simulink library "Px4Library"  (R2015b)
settings: Solver=VariableStepAuto  StartTime=0.0  StopTime=10.0  RelTol=1e-3
undefined symbols (not defined in the file): armed, ctrl_state, INIT_PARAM_VECTOR, mpc_att_sp, mpc_ctrl_state, mpc_manual, mpc_pos_sp_triplet, mpc_vehicle_land_detected, mpc_vehicle_status, v_att_sp, v_control_mode
libraries: simulink x4
(part 7 of 7)

== matlab function Px4Library/attitude_estimator_q/attitude_estimator_q ==
  data: time input; selfVecIn input; selfVecOut output; Q_SAMPLING_PERIOD parameter
function selfVecOut  = qMain( time, selfVecIn, Q_SAMPLING_PERIOD )
%#codegen
	self = DecodeSelf( selfVecIn );
	self = AttitudeEstimatorQ( self, time*1e6 + 149988524 );
	selfVecOut = EncodeSelf( self );
end

function self = DecodeSelf( selfVecIn )
	% Variable assignment
	                           self.acc_comp        = selfVecIn(  1);
	                              self.accel        = zeros( 3, 1);
	                              self.accel( 1, 1) = selfVecIn(  2);
	                              self.accel( 2, 1) = selfVecIn(  3);
	                              self.accel( 3, 1) = selfVecIn(  4);
	    self.airspeed.indicated_airspeed_m_s        = selfVecIn(  5);
	                 self.airspeed.timestamp        = selfVecIn(  6);
	                   self.airspeed.updated        = selfVecIn(  7);
	                      self.airspeed_mode        = selfVecIn(  8);
	self.airspeed_sub.indicated_airspeed_m_s        = selfVecIn(  9);
	             self.airspeed_sub.timestamp        = selfVecIn( 10);
	               self.airspeed_sub.updated        = selfVecIn( 11);
	                  self.att_pub.timestamp        = selfVecIn( 12);
	                  self.att_pub.rollspeed        = selfVecIn( 13);
	                 self.att_pub.pitchspeed        = selfVecIn( 14);
	                   self.att_pub.yawspeed        = selfVecIn( 15);
	                          self.att_pub.q        = zeros( 4, 1);
	                          self.att_pub.q( 1, 1) = selfVecIn( 16);
	                          self.att_pub.q( 2, 1) = selfVecIn( 17);
	                          self.att_pub.q( 3, 1) = selfVecIn( 18);
	                          self.att_pub.q( 4, 1) = selfVecIn( 19);
	                           self.bias_max        = selfVecIn( 20);
	                       self.control_task        = selfVecIn( 21);
	           self.ctrl_state_pub.timestamp        = selfVecIn( 22);
	                   self.ctrl_state_pub.q        = zeros( 4, 1);
	                   self.ctrl_state_pub.q( 1, 1) = selfVecIn( 23);
	                   self.ctrl_state_pub.q( 2, 1) = selfVecIn( 24);
	                   self.ctrl_state_pub.q( 3, 1) = selfVecIn( 25);
	                   self.ctrl_state_pub.q( 4, 1) = selfVecIn( 26);
	               self.ctrl_state_pub.x_acc        = selfVecIn( 27);
	               self.ctrl_state_pub.y_acc        = selfVecIn( 28);
	               self.ctrl_state_pub.z_acc        = selfVecIn( 29);
	           self.ctrl_state_pub.roll_rate        = selfVecIn( 30);
	          self.ctrl_state_pub.pitch_rate        = selfVecIn( 31);
	            self.ctrl_state_pub.yaw_rate        = selfVecIn( 32);
	      self.ctrl_state_pub.roll_rate_bias        = selfVecIn( 33);
	     self.ctrl_state_pub.pitch_rate_bias        = selfVecIn( 34);
	       self.ctrl_state_pub.yaw_rate_bias        = selfVecIn( 35);
	      self.ctrl_state_pub.airspeed_valid        = selfVecIn( 36);
	            self.ctrl_state_pub.airspeed        = selfVecIn( 37);
	                          self.data_good        = selfVecIn( 38);
	                             self.dt_max        = selfVecIn( 39);
	                       self.ext_hdg_good        = selfVecIn( 40);
	                       self.ext_hdg_mode        = selfVecIn( 41);
	             self.global_pos_sub.updated        = selfVecIn( 42);
	                 self.global_pos_sub.eph        = selfVecIn( 43);
	                 self.global_pos_sub.lat        = selfVecIn( 44);
	                 self.global_pos_sub.lon        = selfVecIn( 45);
	           self.global_pos_sub.timestamp        = selfVecIn( 46);
	               self.global_pos_sub.vel_d        = selfVecIn( 47);
	               self.global_pos_sub.vel_e        = selfVecIn( 48);
	               self.global_pos_sub.vel_n        = selfVecIn( 49);
	                       self.gpos.updated        = selfVecIn( 50);
	                           self.gpos.eph        = selfVecIn( 51);
	                           self.gpos.lat        = selfVecIn( 52);
	                           self.gpos.lon        = selfVecIn( 53);
	                     self.gpos.timestamp        = selfVecIn( 54);
	                         self.gpos.vel_d        = selfVecIn( 55);
	                         self.gpos.vel_e        = selfVecIn( 56);
	                         self.gpos.vel_n        = selfVecIn( 57);
	                               self.gyro        = zeros( 3, 1);
	                               self.gyro( 1, 1) = selfVecIn( 58);
	                               self.gyro( 2, 1) = selfVecIn( 59);
	                               self.gyro( 3, 1) = selfVecIn( 60);
	                          self.gyro_bias        = zeros( 3, 1);
	                          self.gyro_bias( 1, 1) = selfVecIn( 61);
	                          self.gyro_bias( 2, 1) = selfVecIn( 62);
	                          self.gyro_bias( 3, 1) = selfVecIn( 63);
	                  self.hrt_absolute_time        = selfVecIn( 64);
	                             self.inited        = selfVecIn( 65);
	             self.lp_accel_x.cutoff_freq        = selfVecIn( 66);
	                      self.lp_accel_x.b0        = selfVecIn( 67);
	                      self.lp_accel_x.b1        = selfVecIn( 68);
	                      self.lp_accel_x.b2        = selfVecIn( 69);
	                      self.lp_accel_x.a1        = selfVecIn( 70);
	                      self.lp_accel_x.a2        = selfVecIn( 71);
	         self.lp_accel_x.delay_element_0        = selfVecIn( 72);
	         self.lp_accel_x.delay_element_1        = selfVecIn( 73);
	         self.lp_accel_x.delay_element_2        = selfVecIn( 74);
	             self.lp_accel_y.cutoff_freq        = selfVecIn( 75);
	                      self.lp_accel_y.b0        = selfVecIn( 76);
	                      self.lp_accel_y.b1        = selfVecIn( 77);
	                      self.lp_accel_y.b2        = selfVecIn( 78);
	                      self.lp_accel_y.a1        = selfVecIn( 79);
	                      self.lp_accel_y.a2        = selfVecIn( 80);
	         self.lp_accel_y.delay_element_0        = selfVecIn( 81);
	         self.lp_accel_y.delay_element_1        = selfVecIn( 82);
	         self.lp_accel_y.delay_element_2        = selfVecIn( 83);
	             self.lp_accel_z.cutoff_freq        = selfVecIn( 84);
	                      self.lp_accel_z.b0        = selfVecIn( 85);
	                      self.lp_accel_z.b1        = selfVecIn( 86);
	                      self.lp_accel_z.b2        = selfVecIn( 87);
	                      self.lp_accel_z.a1        = selfVecIn( 88);
	                      self.lp_accel_z.a2        = selfVecIn( 89);
	         self.lp_accel_z.delay_element_0        = selfVecIn( 90);
	         self.lp_accel_z.delay_element_1        = selfVecIn( 91);
	         self.lp_accel_z.delay_element_2        = selfVecIn( 92);
	              self.lp_gyro_x.cutoff_freq        = selfVecIn( 93);
	                       self.lp_gyro_x.b0        = selfVecIn( 94);
	                       self.lp_gyro_x.b1        = selfVecIn( 95);
	                       self.lp_gyro_x.b2        = selfVecIn( 96);
	                       self.lp_gyro_x.a1        = selfVecIn( 97);
	                       self.lp_gyro_x.a2        = selfVecIn( 98);
	          self.lp_gyro_x.delay_element_0        = selfVecIn( 99);
	          self.lp_gyro_x.delay_element_1        = selfVecIn(100);
	          self.lp_gyro_x.delay_element_2        = selfVecIn(101);
	              self.lp_gyro_y.cutoff_freq        = selfVecIn(102);
	                       self.lp_gyro_y.b0        = selfVecIn(103);
	                       self.lp_gyro_y.b1        = selfVecIn(104);
	                       self.lp_gyro_y.b2        = selfVecIn(105);
	                       self.lp_gyro_y.a1        = selfVecIn(106);
	                       self.lp_gyro_y.a2        = selfVecIn(107);
	          self.lp_gyro_y.delay_element_0        = selfVecIn(108);
	          self.lp_gyro_y.delay_element_1        = selfVecIn(109);
	          self.lp_gyro_y.delay_element_2        = selfVecIn(110);
	              self.lp_gyro_z.cutoff_freq        = selfVecIn(111);
	                       self.lp_gyro_z.b0        = selfVecIn(112);
	                       self.lp_gyro_z.b1        = selfVecIn(113);
	                       self.lp_gyro_z.b2        = selfVecIn(114);
	                       self.lp_gyro_z.a1        = selfVecIn(115);
	                       self.lp_gyro_z.a2        = selfVecIn(116);
	          self.lp_gyro_z.delay_element_0        = selfVecIn(117);
	          self.lp_gyro_z.delay_element_1        = selfVecIn(118);
	          self.lp_gyro_z.delay_element_2        = selfVecIn(119);
	                                self.mag        = zeros( 3, 1);
	                                self.mag( 1, 1) = selfVecIn(120);
	                                self.mag( 2, 1) = selfVecIn(121);
	                                self.mag( 3, 1) = selfVecIn(122);
	                           self.mag_decl        = selfVecIn(123);
	                      self.mag_decl_auto        = selfVecIn(124);
	                    self.mavlink_log_pub        = selfVecIn(125);
	                      self.mocap.updated        = selfVecIn(126);
	                            self.mocap.q        = zeros( 4, 1);
	                            self.mocap.q( 1, 1) = selfVecIn(127);
	                            self.mocap.q( 2, 1) = selfVecIn(128);
	                            self.mocap.q( 3, 1) = selfVecIn(129);
	                            self.mocap.q( 4, 1) = selfVecIn(130);
	                    self.mocap.timestamp        = selfVecIn(131);
	                          self.mocap_hdg        = zeros( 3, 1);
	                          self.mocap_hdg( 1, 1) = selfVecIn(132);
	                          self.mocap_hdg( 2, 1) = selfVecIn(133);
	                          self.mocap_hdg( 3, 1) = selfVecIn(134);
	                  self.mocap_sub.updated        = selfVecIn(135);
	                        self.mocap_sub.q        = zeros( 4, 1);
	                        self.mocap_sub.q( 1, 1) = selfVecIn(136);
	                        self.mocap_sub.q( 2, 1) = selfVecIn(137);
	                        self.mocap_sub.q( 3, 1) = selfVecIn(138);
	                        self.mocap_sub.q( 4, 1) = selfVecIn(139);
	                self.mocap_sub.timestamp        = selfVecIn(140);
	                 self.params_sub.updated        = selfVecIn(141);
	                            self.pos_acc        = zeros( 3, 1);
	                            self.pos_acc( 1, 1) = selfVecIn(142);
	                            self.pos_acc( 2, 1) = selfVecIn(143);
	                            self.pos_acc( 3, 1) = selfVecIn(144);
	                                  self.q        = zeros( 4, 1);
	                                  self.q( 1, 1) = selfVecIn(145);
	                                  self.q( 2, 1) = selfVecIn(146);
	                                  self.q( 3, 1) = selfVecIn(147);
	                                  self.q( 4, 1) = selfVecIn(148);
	                           self.ran_once        = selfVecIn(149);
	                              self.rates        = zeros( 3, 1);
	                              self.rates( 1, 1) = selfVecIn(150);
	                              self.rates( 2, 1) = selfVecIn(151);
	                              self.rates( 3, 1) = selfVecIn(152);
	                self.sensors_sub.updated        = selfVecIn(153);
	              self.sensors_sub.timestamp        = selfVecIn(154);
	               self.sensors_sub.gyro_rad        = zeros( 3, 1);
	               self.sensors_sub.gyro_rad( 1, 1) = selfVecIn(155);
	               self.sensors_sub.gyro_rad( 2, 1) = selfVecIn(156);
	               self.sensors_sub.gyro_rad( 3, 1) = selfVecIn(157);
	     self.sensors_sub.accelerometer_m_s2        = zeros( 3, 1);
	     self.sensors_sub.accelerometer_m_s2( 1, 1) = selfVecIn(158);
	     self.sensors_sub.accelerometer_m_s2( 2, 1) = selfVecIn(159);
	     self.sensors_sub.accelerometer_m_s2( 3, 1) = selfVecIn(160);
	self.sensors_sub.accelerometer_timestamp_relative        = selfVecIn(161);
	        self.sensors_sub.magnetometer_ga        = zeros( 3, 1);
	        self.sensors_sub.magnetometer_ga( 1, 1) = selfVecIn(162);
	        self.sensors_sub.magnetometer_ga( 2, 1) = selfVecIn(163);
	        self.sensors_sub.magnetometer_ga( 3, 1) = selfVecIn(164);
	self.sensors_sub.magnetometer_timestamp_relative        = selfVecIn(165);
	                           self.vel_prev        = zeros( 3, 1);
	                           self.vel_prev( 1, 1) = selfVecIn(166);
	                           self.vel_prev( 2, 1) = selfVecIn(167);
	                           self.vel_prev( 3, 1) = selfVecIn(168);
	                         self.vel_prev_t        = selfVecIn(169);
	                     self.vision.updated        = selfVecIn(170);
	                           self.vision.q        = zeros( 4, 1);
	                           self.vision.q( 1, 1) = selfVecIn(171);
	                           self.vision.q( 2, 1) = selfVecIn(172);
	                           self.vision.q( 3, 1) = selfVecIn(173);
	                           self.vision.q( 4, 1) = selfVecIn(174);
	                   self.vision.timestamp        = selfVecIn(175);
	                         self.vision_hdg        = zeros( 3, 1);
	                         self.vision_hdg( 1, 1) = selfVecIn(176);
	                         self.vision_hdg( 2, 1) = selfVecIn(177);
	                         self.vision_hdg( 3, 1) = selfVecIn(178);
	                 self.vision_sub.updated        = selfVecIn(179);
	                       self.vision_sub.q        = zeros( 4, 1);
	                       self.vision_sub.q( 1, 1) = selfVecIn(180);
	                       self.vision_sub.q( 2, 1) = selfVecIn(181);
	                       self.vision_sub.q( 3, 1) = selfVecIn(182);
	                       self.vision_sub.q( 4, 1) = selfVecIn(183);
	               self.vision_sub.timestamp        = selfVecIn(184);
	                            self.w_accel        = selfVecIn(185);
	                          self.w_ext_hdg        = selfVecIn(186);
	                        self.w_gyro_bias        = selfVecIn(187);
	                              self.w_mag        = selfVecIn(188);
	                                self.now        = selfVecIn(189);
	                          self.last_time        = selfVecIn(190);
end

function selfVecOut = EncodeSelf( self )
	% Variable assignment
	selfVecOut = zeros(190, 1);
	selfVecOut(  1) =                            self.acc_comp( 1, 1);
	selfVecOut(  2) =                               self.accel( 1, 1);
	selfVecOut(  3) =                               self.accel( 2, 1);
	selfVecOut(  4) =                               self.accel( 3, 1);
	selfVecOut(  5) =     self.airspeed.indicated_airspeed_m_s( 1, 1);
	selfVecOut(  6) =                  self.airspeed.timestamp( 1, 1);
	selfVecOut(  7) =                    self.airspeed.updated( 1, 1);
	selfVecOut(  8) =                       self.airspeed_mode( 1, 1);
	selfVecOut(  9) = self.airspeed_sub.indicated_airspeed_m_s( 1, 1);
	selfVecOut( 10) =              self.airspeed_sub.timestamp( 1, 1);
	selfVecOut( 11) =                self.airspeed_sub.updated( 1, 1);
	selfVecOut( 12) =                   self.att_pub.timestamp( 1, 1);
	selfVecOut( 13) =                   self.att_pub.rollspeed( 1, 1);
	selfVecOut( 14) =                  self.att_pub.pitchspeed( 1, 1);
	selfVecOut( 15) =                    self.att_pub.yawspeed( 1, 1);
	selfVecOut( 16) =                           self.att_pub.q( 1, 1);
	selfVecOut( 17) =                           self.att_pub.q( 2, 1);
	selfVecOut( 18) =                           self.att_pub.q( 3, 1);
	selfVecOut( 19) =                           self.att_pub.q( 4, 1);
	selfVecOut( 20) =                            self.bias_max( 1, 1);
	selfVecOut( 21) =                        self.control_task( 1, 1);
	selfVecOut( 22) =            self.ctrl_state_pub.timestamp( 1, 1);
	selfVecOut( 23) =                    self.ctrl_state_pub.q( 1, 1);
	selfVecOut( 24) =                    self.ctrl_state_pub.q( 2, 1);
	selfVecOut( 25) =                    self.ctrl_state_pub.q( 3, 1);
	selfVecOut( 26) =                    self.ctrl_state_pub.q( 4, 1);
	selfVecOut( 27) =                self.ctrl_state_pub.x_acc( 1, 1);
	selfVecOut( 28) =                self.ctrl_state_pub.y_acc( 1, 1);
	selfVecOut( 29) =                self.ctrl_state_pub.z_acc( 1, 1);
	selfVecOut( 30) =            self.ctrl_state_pub.roll_rate( 1, 1);
	selfVecOut( 31) =           self.ctrl_state_pub.pitch_rate( 1, 1);
	selfVecOut( 32) =             self.ctrl_state_pub.yaw_rate( 1, 1);
	selfVecOut( 33) =       self.ctrl_state_pub.roll_rate_bias( 1, 1);
	selfVecOut( 34) =      self.ctrl_state_pub.pitch_rate_bias( 1, 1);
	selfVecOut( 35) =        self.ctrl_state_pub.yaw_rate_bias( 1, 1);
	selfVecOut( 36) =       self.ctrl_state_pub.airspeed_valid( 1, 1);
	selfVecOut( 37) =             self.ctrl_state_pub.airspeed( 1, 1);
	selfVecOut( 38) =                           self.data_good( 1, 1);
	selfVecOut( 39) =                              self.dt_max( 1, 1);
	selfVecOut( 40) =                        self.ext_hdg_good( 1, 1);
	selfVecOut( 41) =                        self.ext_hdg_mode( 1, 1);
	selfVecOut( 42) =              self.global_pos_sub.updated( 1, 1);
	selfVecOut( 43) =                  self.global_pos_sub.eph( 1, 1);
	selfVecOut( 44) =                  self.global_pos_sub.lat( 1, 1);
	selfVecOut( 45) =                  self.global_pos_sub.lon( 1, 1);
	selfVecOut( 46) =            self.global_pos_sub.timestamp( 1, 1);
	selfVecOut( 47) =                self.global_pos_sub.vel_d( 1, 1);
	selfVecOut( 48) =                self.global_pos_sub.vel_e( 1, 1);
	selfVecOut( 49) =                self.global_pos_sub.vel_n( 1, 1);
	selfVecOut( 50) =                        self.gpos.updated( 1, 1);
	selfVecOut( 51) =                            self.gpos.eph( 1, 1);
	selfVecOut( 52) =                            self.gpos.lat( 1, 1);
	selfVecOut( 53) =                            self.gpos.lon( 1, 1);
	selfVecOut( 54) =                      self.gpos.timestamp( 1, 1);
	selfVecOut( 55) =                          self.gpos.vel_d( 1, 1);
	selfVecOut( 56) =                          self.gpos.vel_e( 1, 1);
	selfVecOut( 57) =                          self.gpos.vel_n( 1, 1);
	selfVecOut( 58) =                                self.gyro( 1, 1);
	selfVecOut( 59) =                                self.gyro( 2, 1);
	selfVecOut( 60) =                                self.gyro( 3, 1);
	selfVecOut( 61) =                           self.gyro_bias( 1, 1);
	selfVecOut( 62) =                           self.gyro_bias( 2, 1);
	selfVecOut( 63) =                           self.gyro_bias( 3, 1);
	selfVecOut( 64) =                   self.hrt_absolute_time( 1, 1);
	selfVecOut( 65) =                              self.inited( 1, 1);
	selfVecOut( 66) =              self.lp_accel_x.cutoff_freq( 1, 1);
	selfVecOut( 67) =                       self.lp_accel_x.b0( 1, 1);
	selfVecOut( 68) =                       self.lp_accel_x.b1( 1, 1);
	selfVecOut( 69) =                       self.lp_accel_x.b2( 1, 1);
	selfVecOut( 70) =                       self.lp_accel_x.a1( 1, 1);
	selfVecOut( 71) =                       self.lp_accel_x.a2( 1, 1);
	selfVecOut( 72) =          self.lp_accel_x.delay_element_0( 1, 1);
	selfVecOut( 73) =          self.lp_accel_x.delay_element_1( 1, 1);
	selfVecOut( 74) =          self.lp_accel_x.delay_element_2( 1, 1);
	selfVecOut( 75) =              self.lp_accel_y.cutoff_freq( 1, 1);
	selfVecOut( 76) =                       self.lp_accel_y.b0( 1, 1);
	selfVecOut( 77) =                       self.lp_accel_y.b1( 1, 1);
	selfVecOut( 78) =                       self.lp_accel_y.b2( 1, 1);
	selfVecOut( 79) =                       self.lp_accel_y.a1( 1, 1);
	selfVecOut( 80) =                       self.lp_accel_y.a2( 1, 1);
	selfVecOut( 81) =          self.lp_accel_y.delay_element_0( 1, 1);
	selfVecOut( 82) =          self.lp_accel_y.delay_element_1( 1, 1);
	selfVecOut( 83) =          self.lp_accel_y.delay_element_2( 1, 1);
	selfVecOut( 84) =              self.lp_accel_z.cutoff_freq( 1, 1);
	selfVecOut( 85) =                       self.lp_accel_z.b0( 1, 1);
	selfVecOut( 86) =                       self.lp_accel_z.b1( 1, 1);
	selfVecOut( 87) =                       self.lp_accel_z.b2( 1, 1);
	selfVecOut( 88) =                       self.lp_accel_z.a1( 1, 1);
	selfVecOut( 89) =                       self.lp_accel_z.a2( 1, 1);
	selfVecOut( 90) =          self.lp_accel_z.delay_element_0( 1, 1);
	selfVecOut( 91) =          self.lp_accel_z.delay_element_1( 1, 1);
	selfVecOut( 92) =          self.lp_accel_z.delay_element_2( 1, 1);
	selfVecOut( 93) =               self.lp_gyro_x.cutoff_freq( 1, 1);
	selfVecOut( 94) =                        self.lp_gyro_x.b0( 1, 1);
	selfVecOut( 95) =                        self.lp_gyro_x.b1( 1, 1);
	selfVecOut( 96) =                        self.lp_gyro_x.b2( 1, 1);
	selfVecOut( 97) =                        self.lp_gyro_x.a1( 1, 1);
	selfVecOut( 98) =                        self.lp_gyro_x.a2( 1, 1);
	selfVecOut( 99) =           self.lp_gyro_x.delay_element_0( 1, 1);
	selfVecOut(100) =           self.lp_gyro_x.delay_element_1( 1, 1);
	selfVecOut(101) =           self.lp_gyro_x.delay_element_2( 1, 1);
	selfVecOut(102) =               self.lp_gyro_y.cutoff_freq( 1, 1);
	selfVecOut(103) =                        self.lp_gyro_y.b0( 1, 1);
	selfVecOut(104) =                        self.lp_gyro_y.b1( 1, 1);
	selfVecOut(105) =                        self.lp_gyro_y.b2( 1, 1);
	selfVecOut(106) =                        self.lp_gyro_y.a1( 1, 1);
	selfVecOut(107) =                        self.lp_gyro_y.a2( 1, 1);
	selfVecOut(108) =           self.lp_gyro_y.delay_element_0( 1, 1);
	selfVecOut(109) =           self.lp_gyro_y.delay_element_1( 1, 1);
	selfVecOut(110) =           self.lp_gyro_y.delay_element_2( 1, 1);
	selfVecOut(111) =               self.lp_gyro_z.cutoff_freq( 1, 1);
	selfVecOut(112) =                        self.lp_gyro_z.b0( 1, 1);
	selfVecOut(113) =                        self.lp_gyro_z.b1( 1, 1);
	selfVecOut(114) =                        self.lp_gyro_z.b2( 1, 1);
	selfVecOut(115) =                        self.lp_gyro_z.a1( 1, 1);
	selfVecOut(116) =                        self.lp_gyro_z.a2( 1, 1);
	selfVecOut(117) =           self.lp_gyro_z.delay_element_0( 1, 1);
	selfVecOut(118) =           self.lp_gyro_z.delay_element_1( 1, 1);
	selfVecOut(119) =           self.lp_gyro_z.delay_element_2( 1, 1);
	selfVecOut(120) =                                 self.mag( 1, 1);
	selfVecOut(121) =                                 self.mag( 2, 1);
	selfVecOut(122) =                                 self.mag( 3, 1);
	selfVecOut(123) =                            self.mag_decl( 1, 1);
	selfVecOut(124) =                       self.mag_decl_auto( 1, 1);
	selfVecOut(125) =                     self.mavlink_log_pub( 1, 1);
	selfVecOut(126) =                       self.mocap.updated( 1, 1);
	selfVecOut(127) =                             self.mocap.q( 1, 1);
	selfVecOut(128) =                             self.mocap.q( 2, 1);
	selfVecOut(129) =                             self.mocap.q( 3, 1);
	selfVecOut(130) =                             self.mocap.q( 4, 1);
	selfVecOut(131) =                     self.mocap.timestamp( 1, 1);
	selfVecOut(132) =                           self.mocap_hdg( 1, 1);
	selfVecOut(133) =                           self.mocap_hdg( 2, 1);
	selfVecOut(134) =                           self.mocap_hdg( 3, 1);
	selfVecOut(135) =                   self.mocap_sub.updated( 1, 1);
	selfVecOut(136) =                         self.mocap_sub.q( 1, 1);
	selfVecOut(137) =                         self.mocap_sub.q( 2, 1);
	selfVecOut(138) =                         self.mocap_sub.q( 3, 1);
	selfVecOut(139) =                         self.mocap_sub.q( 4, 1);
	selfVecOut(140) =                 self.mocap_sub.timestamp( 1, 1);
	selfVecOut(141) =                  self.params_sub.updated( 1, 1);
	selfVecOut(142) =                             self.pos_acc( 1, 1);
	selfVecOut(143) =                             self.pos_acc( 2, 1);
	selfVecOut(144) =                             self.pos_acc( 3, 1);
	selfVecOut(145) =                                   self.q( 1, 1);
	selfVecOut(146) =                                   self.q( 2, 1);
	selfVecOut(147) =                                   self.q( 3, 1);
	selfVecOut(148) =                                   self.q( 4, 1);
	selfVecOut(149) =                            self.ran_once( 1, 1);
	selfVecOut(150) =                               self.rates( 1, 1);
	selfVecOut(151) =                               self.rates( 2, 1);
	selfVecOut(152) =                               self.rates( 3, 1);
	selfVecOut(153) =                 self.sensors_sub.updated( 1, 1);
	selfVecOut(154) =               self.sensors_sub.timestamp( 1, 1);
	selfVecOut(155) =                self.sensors_sub.gyro_rad( 1, 1);
	selfVecOut(156) =                self.sensors_sub.gyro_rad( 2, 1);
	selfVecOut(157) =                self.sensors_sub.gyro_rad( 3, 1);
	selfVecOut(158) =      self.sensors_sub.accelerometer_m_s2( 1, 1);
	selfVecOut(159) =      self.sensors_sub.accelerometer_m_s2( 2, 1);
	selfVecOut(160) =      self.sensors_sub.accelerometer_m_s2( 3, 1);
	selfVecOut(161) = self.sensors_sub.accelerometer_timestamp_relative( 1, 1);
	selfVecOut(162) =         self.sensors_sub.magnetometer_ga( 1, 1);
	selfVecOut(163) =         self.sensors_sub.magnetometer_ga( 2, 1);
	selfVecOut(164) =         self.sensors_sub.magnetometer_ga( 3, 1);
	selfVecOut(165) = self.sensors_sub.magnetometer_timestamp_relative( 1, 1);
	selfVecOut(166) =                            self.vel_prev( 1, 1);
	selfVecOut(167) =                            self.vel_prev( 2, 1);
	selfVecOut(168) =                            self.vel_prev( 3, 1);
	selfVecOut(169) =                          self.vel_prev_t( 1, 1);
	selfVecOut(170) =                      self.vision.updated( 1, 1);
	selfVecOut(171) =                            self.vision.q( 1, 1);
	selfVecOut(172) =                            self.vision.q( 2, 1);
	selfVecOut(173) =                            self.vision.q( 3, 1);
	selfVecOut(174) =                            self.vision.q( 4, 1);
	selfVecOut(175) =                    self.vision.timestamp( 1, 1);
	selfVecOut(176) =                          self.vision_hdg( 1, 1);
	selfVecOut(177) =                          self.vision_hdg( 2, 1);
	selfVecOut(178) =                          self.vision_hdg( 3, 1);
	selfVecOut(179) =                  self.vision_sub.updated( 1, 1);
	selfVecOut(180) =                        self.vision_sub.q( 1, 1);
	selfVecOut(181) =                        self.vision_sub.q( 2, 1);
	selfVecOut(182) =                        self.vision_sub.q( 3, 1);
	selfVecOut(183) =                        self.vision_sub.q( 4, 1);
	selfVecOut(184) =                self.vision_sub.timestamp( 1, 1);
	selfVecOut(185) =                             self.w_accel( 1, 1);
	selfVecOut(186) =                           self.w_ext_hdg( 1, 1);
	selfVecOut(187) =                         self.w_gyro_bias( 1, 1);
	selfVecOut(188) =                               self.w_mag( 1, 1);
	selfVecOut(189) =                                 self.now( 1, 1);
	selfVecOut(190) =                           self.last_time( 1, 1);
end

% %***************************************************************************
%  *
%  *   Copyright (c) 2015 PX4 Development Team. All rights reserved.
%  *
%  * Redistribution and use in source and binary forms, with or without
%  * modification, are permitted provided that the following conditions
%  * are met:
%  *
%  * 1. Redistributions of source code must retain the above copyright
%  *    notice, this list of conditions and the following disclaimer.
%  * 2. Redistributions in binary form must reproduce the above copyright
%  *    notice, this list of conditions and the following disclaimer in
%  *    the documentation and/or other materials provided with the
%  *    distribution.
%  * 3. Neither the name PX4 nor the names of its contributors may be
%  *    used to endorse or promote products derived from this software
%  *    without specific prior written permission.
%  *
%  * THIS SOFTWARE IS PROVIDED BY THE COPYRIGHT HOLDERS AND CONTRIBUTORS
%  * 'AS IS' AND ANY EXPRESS OR IMPLIED WARRANTIES, INCLUDING, BUT NOT
%  * LIMITED TO, THE IMPLIED WARRANTIES OF MERCHANTABILITY AND FITNESS
%  * FOR A PARTICULAR PURPOSE ARE DISCLAIMED. IN NO EVENT SHALL THE
%  * COPYRIGHT OWNER OR CONTRIBUTORS BE LIABLE FOR ANY DIRECT, INDIRECT,
%  * INCIDENTAL, SPECIAL, EXEMPLARY, OR CONSEQUENTIAL DAMAGES (INCLUDING,
%  * BUT NOT LIMITED TO, PROCUREMENT OF SUBSTITUTE GOODS OR SERVICES; LOSS
%  * OF USE, DATA, OR PROFITS; OR BUSINESS INTERRUPTION) HOWEVER CAUSED
%  * AND ON ANY THEORY OF LIABILITY, WHETHER IN CONTRACT, STRICT
%  * LIABILITY, OR TORT (INCLUDING NEGLIGENCE OR OTHERWISE) ARISING IN
%  * ANY WAY OUT OF THE USE OF THIS SOFTWARE, EVEN IF ADVISED OF THE
%  * POSSIBILITY OF SUCH DAMAGE.
%  *
%  ****************************************************************************/

% %
%  * @file attitude_estimator_q_main.cpp
%  *
%  * Attitude estimator (quaternion based)
%  *
%  * @author Anton Babushkin <anton.babushkin@me.com>
% 

% #include <px4_config.h>
% #include <px4_posix.h>
% #include <px4_tasks.h>
% #include <unistd.h>
% #include <stdlib.h>
% #include <stdio.h>
% #include <stdbool.h>
% #include <poll.h>
% #include <fcntl.h>
% #include <float.h>
% #include <errno.h>
% #include <limits.h>
% #include <math.h>
% #include <uORB/uORB.h>
% #include <uORB/topics/sensor_combined.h>
% #include <uORB/topics/vehicle_attitude.h>
% #include <uORB/topics/control_state.h>
% #include <uORB/topics/vehicle_control_mode.h>
% #include <uORB/topics/vehicle_global_position.h>
% #include <uORB/topics/att_pos_mocap.h>
% #include <uORB/topics/airspeed.h>
% #include <uORB/topics/parameter_update.h>
% #include <uORB/topics/estimator_status.h>
% #include <drivers/drv_hrt.h>
% 
% #include <mathlib/mathlib.h>
% #include <mathlib/math/filter/LowPassFilter2p.hpp>
% #include <lib/geo/geo.h>
% 
% #include <systemlib/param/param.h>
% #include <systemlib/perf_counter.h>
% #include <systemlib/err.h>
% #include <systemlib/mavlink_log.h>
% 
% extern 'C' self._EXPORT int attitude_estimator_q_main(int argc, char *argv[]);
% 
% using math::Vector;
% using math::Matrix;
% using math::Quaternion;
% 
% class AttitudeEstimatorQ;
% 
% namespace attitude_estimator_q
% 
% AttitudeEstimatorQ *instance;
% }


% class AttitudeEstimatorQ
% 
% public:
% 	%*
% 	 * Constructor
% 	
% 	AttitudeEstimatorQ();
% 
% 	%*
% 	 * Destructor, also kills task.
% 	
% 	~AttitudeEstimatorQ();
% 
% 	%*
% 	 * Start task.
% 	 *
% 	 * @return		1 on success.
% 	
% 	int		start();
% 
% 	static void	task_main_trampoline(int argc, char *argv[]);
% 
% 	void		task_main();
% 
% 	void		print();
% 
% private:
% 	static constexpr float self.dt_max = 0.02;
% 	bool		self.task_should_exit = 0;		%*< if 1, task should exit
% 	int		self.control_task = -1;			%*< task handle for task
% 
% 	int		self.sensors_sub = -1;
% 	int		self.params_sub = -1;
% 	int		self.vision_sub = -1;
% 	int		self.mocap_sub = -1;
% 	int		self.airspeed_sub = -1;
% 	int		self.global_pos_sub = -1;
% 	orb_advert_t	self.att_pub = nullptr;
% 	orb_advert_t	self.ctrl_state_pub = nullptr;
% 	orb_advert_t	self.est_state_pub = nullptr;
% 
% 	struct 
% 		param_t	w_acc;
% 		param_t	w_mag;
% 		param_t	w_ext_hdg;
% 		param_t	w_gyro_bias;
% 		param_t	mag_decl;
% 		param_t	mag_decl_auto;
% 		param_t	acc_comp;
% 		param_t	bias_max;
% 		param_t	ext_hdg_mode;
% 		param_t airspeed_mode;
% 	}		self.params_handles;		%*< handles for interesting parameters
% 
% 	float		self.w_accel = 0.0;
% 	float		self.w_mag = 0.0;
% 	float		self.w_ext_hdg = 0.0;
% 	float		self.w_gyro_bias = 0.0;
% 	float		self.mag_decl = 0.0;
% 	bool		self.mag_decl_auto = 0;
% 	bool		self.acc_comp = 0;
% 	float		self.bias_max = 0.0;
% 	int		self.ext_hdg_mode = 0;
% 	int 	self.airspeed_mode = 0;
% 
% 	Vector<3>	self.gyro;
% 	Vector<3>	self.accel;
% 	Vector<3>	self.mag;
% 
% 	vehicle_attitude_s self.vision = {};
% 	Vector<3>	self.vision_hdg;
% 
% 	att_pos_mocap_s self.mocap = {};
% 	Vector<3>	self.mocap_hdg;
% 
% 	airspeed_s self.airspeed = {};
% 
% 	Quaternion	self.q;
% 	Vector<3>	self.rates;
% 	Vector<3>	self.gyro_bias;
% 
% 	vehicle_global_position_s self.gpos = {};
% 	Vector<3>	self.vel_prev;
% 	Vector<3>	self.pos_acc;
% 
% 	% Low pass filter for accel/gyro
% 	math::LowPassFilter2p self.lp_accel_x;
% 	math::LowPassFilter2p self.lp_accel_y;
% 	math::LowPassFilter2p self.lp_accel_z;
% 	math::LowPassFilter2p self.lp_gyro_x;
% 	math::LowPassFilter2p self.lp_gyro_y;
% 	math::LowPassFilter2p self.lp_gyro_z;
% 
% 	hrt_abstime self.vel_prev_t = 0;
% 
% 	bool		self.inited = 0;
% 	bool		self.data_good = 0;
% 	bool		self.ext_hdg_good = 0;
% 
% 	orb_advert_t	self.mavlink_log_pub = nullptr;
% 
% 	void update_parameters(bool force);
% 
% 	int update_subscriptions();
% 
% 	bool init();
% 
% 	bool update(float dt);
% 
% 	% Update magnetic declination (in rads) immediately changing yaw rotation
% 	void update_mag_declination(float new_declination);
% };


% AttitudeEstimatorQ:: :
function self = AttitudeEstimatorQ( self, timestamp )
% 	self.vel_prev(0, 0, 0),
% 	self.pos_acc(0, 0, 0),
    if (~self.ran_once)
        self.lp_accel_x = lp2p_set_cutoff_frequency( self.lp_accel_x, 250.0, 30.0 );
        self.lp_accel_y = lp2p_set_cutoff_frequency( self.lp_accel_y, 250.0, 30.0 );
        self.lp_accel_z = lp2p_set_cutoff_frequency( self.lp_accel_z, 250.0, 30.0 );
        self.lp_gyro_x = lp2p_set_cutoff_frequency( self.lp_gyro_x, 250.0, 30.0 );
        self.lp_gyro_y = lp2p_set_cutoff_frequency( self.lp_gyro_y, 250.0, 30.0 );
        self.lp_gyro_z = lp2p_set_cutoff_frequency( self.lp_gyro_z, 250.0, 30.0 );
        self.ran_once = 1;
    end
% 	self.params_handles.w_acc		= param_find('ATT_W_ACC');
% 	self.params_handles.w_mag		= param_find('ATT_W_MAG');
% 	self.params_handles.w_ext_hdg	= param_find('ATT_W_EXT_HDG');
% 	self.params_handles.w_gyro_bias	= param_find('ATT_W_GYRO_BIAS');
% 	self.params_handles.mag_decl	= param_find('ATT_MAG_DECL');
% 	self.params_handles.mag_decl_auto	= param_find('ATT_MAG_DECL_A');
% 	self.params_handles.acc_comp	= param_find('ATT_ACC_COMP');
% 	self.params_handles.bias_max	= param_find('ATT_BIAS_MAX');
% 	self.params_handles.ext_hdg_mode	= param_find('ATT_EXT_HDG_M');
% 	self.params_handles.airspeed_mode = param_find('FW_ARSP_MODE');
    self.hrt_absolute_time = timestamp;
    self = task_main( self );
end

%  Destructor, also kills task.
% AttitudeEstimatorQ::~
% function self = self = AttitudeEstimatorQDestructor( self )

% 	if (self.control_task ~= -1) 
% 		% task wakes up every 100ms or so at the longest
% 		self.task_should_exit = 1;

% 		% wait for a second for the task to quit at our request
% 		unsigned i = 0;

% 		do 
% 			% wait 20ms
% 			usleep(20000);

% 			% if we have given up, kill it
% 			if (++i > 50) 
% 				px4_task_delete(self.control_task);
% 				break;
% 			end
% 		end while (self.control_task ~= -1);
% 	end

% 	attitude_estimator_q::instance = nullptr;
% end

% Probably not needed
% int AttitudeEstimatorQ::
% function [ self, output ] = start( self )
% %START
% 	ASSERT(self.control_task == -1);
% 
% 	% start the task
% % 	self.control_task = px4_task_spawn_cmd('attitude_estimator_q', ...
% % 					   SCHED_DEFAULT, ...
% % 					   SCHED_PRIORITY_MAX - 5, ...
% % 					   2000, ...
% % 					   (px4_main_t)&AttitudeEstimatorQ::task_main_trampoline,
% % 					   nullptr);
% 
% 	if (self.control_task < 0) 
% 		warn('task start failed');
% 		output = -errno;
%         return;
% 	end
% 
% 	output = 1;
% end

% void AttitudeEstimatorQ::
% function self = print( self )
% %PRINT
%     % Empty
% end

% void AttitudeEstimatorQ::
% function self = task_main_trampoline( self )
% %TASK_MAIN_TRAMPOLINE
% 	% attitude_estimator_q::instance->
%     self = task_main( self );
% end

% void AttitudeEstimatorQ::
function self = task_main( self )
% ifdef self._PX4_POSIX
%     % All perf_counter_t
% 	self.perf_accel(perf_alloc_once(PC_ELAPSED, 'sim_accel_delay'));
% 	self.perf_mpu(perf_alloc_once(PC_ELAPSED, 'sim_mpu_delay'));
% 	self.perf_mag(perf_alloc_once(PC_ELAPSED, 'sim_mag_delay'));
% endif

    % Subscriptions
% 	self.sensors_sub = orb_subscribe(ORB_ID(sensor_combined));
% 	self.vision_sub = orb_subscribe(ORB_ID(vehicle_vision_attitude));
% 	self.mocap_sub = orb_subscribe(ORB_ID(att_pos_mocap));
% 	self.airspeed_sub = orb_subscribe(ORB_ID(airspeed));
% 	self.params_sub = orb_subscribe(ORB_ID(parameter_update));
% 	self.global_pos_sub = orb_subscribe(ORB_ID(vehicle_global_position));

	% self = update_parameters( self, 1 );

	% hrt_abstime
    % self.last_time = 0;

	% px4_pollfd_struct_t fds[1] = {};
	% fds[0].fd = self.sensors_sub;
	% fds[0].events = POLLIN;

% 	while ( ~self.task_should_exit ) 
		%int
        % ret = px4_poll(fds, 1, 1000);

% 		if (ret < 0) 
% 			% Poll error, sleep and try again
% 			usleep(10000);
% 			% PX4_WARN('Q POLL ERROR');
% 			continue;
% 
% 		elseif (ret == 0) 
% 			% Poll timeout, do nothing
% 			% PX4_WARN('Q POLL TIMEOUT');
% 			continue;
% 		end

% 		self = update_parameters( self, 0 );

		% Update sensors
		% sensor_combined_s sensors ;

		% if (~orb_copy(ORB_ID(sensor_combined), self.sensors_sub, sensors))
        sensors_updated = self.sensors_sub.updated;
        sensors = self.sensors_sub;
        
        if sensors_updated
			% Feed validator with recent sensor data
			if (sensors.timestamp > 0) 
				% Filter gyro signal since it is not fildered in the drivers.
				[self.lp_gyro_x, self.gyro(1)] = lp2p_apply( self.lp_gyro_x, sensors.gyro_rad(1) );
				[self.lp_gyro_y, self.gyro(2)] = lp2p_apply( self.lp_gyro_y, sensors.gyro_rad(2) );
				[self.lp_gyro_z, self.gyro(3)] = lp2p_apply( self.lp_gyro_z, sensors.gyro_rad(3) );
			end

			if ( sensors.accelerometer_timestamp_relative ~= 2147483647 ) % sensor_combined_s.RELATIVE_TIMESTAMP_INVALID ) 
				% Filter accel signal since it is not fildered in the drivers.
				[self.lp_accel_x, self.accel(1)] = lp2p_apply( self.lp_accel_x, sensors.accelerometer_m_s2(1) );
				[self.lp_accel_y, self.accel(2)] = lp2p_apply( self.lp_accel_y, sensors.accelerometer_m_s2(2) );
				[self.lp_accel_z, self.accel(3)] = lp2p_apply( self.lp_accel_z, sensors.accelerometer_m_s2(3) );

				if ( norm(self.accel) < 0.01) 
					% disp('WARNING: degenerate accel~');
					% continue;
                    return;
				end
			end

			if ( sensors.magnetometer_timestamp_relative ~= 2147483647 ) % sensor_combined_s.RELATIVE_TIMESTAMP_INVALID ) 
				self.mag(1) = sensors.magnetometer_ga(1);
				self.mag(2) = sensors.magnetometer_ga(2);
				self.mag(3) = sensors.magnetometer_ga(3);

				if ( norm(self.mag) < 0.01 ) 
					% disp('WARNING: degenerate mag~');
					% continue;
                    return;
				end
			end

			self.data_good = 1;
        end

		% Update vision and motion capture heading
        % bool
		vision_updated = self.vision_sub.updated;
		% orb_check(self.vision_sub, vision_updated);

		% bool
        mocap_updated = self.mocap_sub.updated;
		% orb_check(self.mocap_sub, mocap_updated);

		if (vision_updated) 
			% orb_copy(ORB_ID(vehicle_vision_attitude), self.vision_sub, &self.vision);
            self.vision = self.vision_sub;
			% math::Quaternion
            q = self.vision.q;

			% math::Matrix<3, 3>
            Rvis = quat_to_dcm( q );
			% math::Vector<3>
            v = [1.0; 0.0; 0.4];

			% Rvis is Rwr (robot respect to world) while v is respect to world.
			% Hence Rvis must be transposed having (Rwr)' * Vw
			% Rrw * Vw = vn. This way we have consistency
			self.vision_hdg = Rvis' * v;
		end

		if (mocap_updated) 
			% orb_copy(ORB_ID(att_pos_mocap), self.mocap_sub, &self.mocap);
            self.mocap = self.mocap_sub;
			% math::Quaternion
            q = self.mocap.q;
			% math::Matrix<3, 3>
            Rmoc = quat_to_dcm( q );

			% math::Vector<3>
            v = [1.0; 0.0; 0.4];

			% Rmoc is Rwr (robot respect to world) while v is respect to world.
			% Hence Rmoc must be transposed having (Rwr)' * Vw
			% Rrw * Vw = vn. This way we have consistency
			self.mocap_hdg = Rmoc' * v;
		end

		% Update airspeed
		% bool
        airspeed_updated = self.airspeed_sub.updated;
		% orb_check(self.airspeed_sub, &airspeed_updated);

		if ( airspeed_updated ) 
			% orb_copy(ORB_ID(airspeed), self.airspeed_sub, &self.airspeed);
            self.airspeed = self.airspeed_sub;
		end

		% Check for timeouts on data
		if (self.ext_hdg_mode == 2) 
			self.ext_hdg_good = double( (self.vision.timestamp > 0) && ( (self.hrt_absolute_time - self.vision.timestamp) < 500000 ) );

		elseif (self.ext_hdg_mode == 3) 
			self.ext_hdg_good = double( (self.mocap.timestamp > 0) && ((self.hrt_absolute_time - self.mocap.timestamp) < 500000) );
		end

		% bool
        gpos_updated = self.global_pos_sub.updated;
		% orb_check(self.global_pos_sub, &gpos_updated);

		if ( gpos_updated ) 
			%orb_copy(ORB_ID(vehicle_global_position), self.global_pos_sub, &self.gpos);
            self.gpos = self.global_pos_sub;

			if ( self.mag_decl_auto && (self.gpos.eph < 20.0) && ((self.hrt_absolute_time - self.gpos.timestamp) < 1000000) ) 
				% set magnetic declination automatically
				self = update_mag_declination( self, ( get_mag_declination(self.gpos.lat, self.gpos.lon) ) * pi / 180 );
			end
		end

		if ( self.acc_comp && ...
             (self.gpos.timestamp ~= 0) && ...
             (self.hrt_absolute_time < (self.gpos.timestamp + 20000)) && ...
             (self.gpos.eph < 5.0) && ...
             self.inited ) 
			% position data is actual
			if (gpos_updated) 
				% Vector<3>
                vel = [self.gpos.vel_n; self.gpos.vel_e; self.gpos.vel_d];

				% velocity updated
				if ( (self.vel_prev_t ~= 0) && (self.gpos.timestamp ~= self.vel_prev_t) )
					% float
                    vel_dt = (self.gpos.timestamp - self.vel_prev_t) / 1000000.0;
					% calculate acceleration in body frame
					self.pos_acc = quat_conjugate_inversed( self.q, (vel - self.vel_prev) / vel_dt);
				end

				self.vel_prev_t = self.gpos.timestamp;
				self.vel_prev = vel;
			end

		else 
			% position data is outdated, reset acceleration
			self.pos_acc = zeros(3, 1);
			self.vel_prev = zeros(3, 1);
			self.vel_prev_t = 0;
		end

		% time from previous iteration
		% hrt_abstime
        self.now = self.hrt_absolute_time;
		% float
        if (self.last_time > 0)
            dt =  (self.now  - self.last_time) / 1000000.0;
        else
            dt = 0.00001;
        end
        
		self.last_time = self.now;

        if ( dt > self.dt_max )
            dt = self.dt_max;
        end
    
        [self, status] = update( self, dt );
        if ( ~status ) 
            % continue;
            return;
        end
        
        %vehicle_attitude_s
        att.timestamp  = sensors.timestamp;
        att.rollspeed  = self.rates(1);
        att.pitchspeed = self.rates(2);
        att.yawspeed   = self.rates(3);
        att.q = [self.q(1); self.q(2); self.q(3); self.q(4)];

        % the instance count is not used here
        % int att_inst;
        % orb_publish_auto(ORB_ID(vehicle_attitude), &self.att_pub, &att, &att_inst, ORB_PRIO_HIGH);
        self.att_pub = att;

        % struct
        % control_state_s ctrl_state = {};

        ctrl_state.timestamp = sensors.timestamp;

        % attitude quaternions for control state
        ctrl_state.q = self.q;

        ctrl_state.x_acc = self.accel(1);
        ctrl_state.y_acc = self.accel(2);
        ctrl_state.z_acc = self.accel(3);

        % attitude rates for control state
        ctrl_state.roll_rate  = self.rates(1);
        ctrl_state.pitch_rate = self.rates(2);
        ctrl_state.yaw_rate   = self.rates(3);

        % TODO get bias estimates from estimator
        ctrl_state.roll_rate_bias = 0.0;
        ctrl_state.pitch_rate_bias = 0.0;
        ctrl_state.yaw_rate_bias = 0.0;

        ctrl_state.airspeed_valid = 0;
        ctrl_state.airspeed = 0;

        if (self.airspeed_mode == 0 ) % control_state_s.AIRSPD_MODE_MEAS) 
            % use measured airspeed
            if (isfinite(self.airspeed.indicated_airspeed_m_s) && ...
                    (self.hrt_absolute_time - self.airspeed.timestamp < 1e6) && ...
                    (self.airspeed.timestamp > 0) ) 
                ctrl_state.airspeed = self.airspeed.indicated_airspeed_m_s;
                ctrl_state.airspeed_valid = 1;
            end
        elseif (self.airspeed_mode == 1 ) % control_state_s.AIRSPD_MODE_EST) 
            % use estimated body velocity as airspeed estimate
            if ( (self.hrt_absolute_time - self.gpos.timestamp) < 1e6) 
                ctrl_state.airspeed = sqrt(self.gpos.vel_n * self.gpos.vel_n + self.gpos.vel_e * self.gpos.vel_e + self.gpos.vel_d * self.gpos.vel_d);
                ctrl_state.airspeed_valid = 1;
            end

        elseif (self.airspeed_mode == 2 ) % control_state_s.AIRSPD_MODE_DISABLED) 
            % do nothing, airspeed has been declared as non-valid above, controllers
            % will handle this assuming always trim airspeed
        end

        % the instance count is not used here
        % int ctrl_inst;
        % publish to control state topic
        % orb_publish_auto(ORB_ID(control_state), &self.ctrl_state_pub, &ctrl_state, &ctrl_inst, ORB_PRIO_HIGH);
        self.ctrl_state_pub = ctrl_state;

        %struct estimator_status_s est = {};

        %est.timestamp = sensors.timestamp;

        % the instance count is not used here
        %int est_inst;
        % publish to control state topic
        % TODO handle attitude states in position estimators instead so we can publish all data at once
        % or we need to enable more thatn just one estimator_status topic
        % orb_publish_auto(ORB_ID(estimator_status), &self.est_state_pub, &est, &est_inst, ORB_PRIO_HIGH);
%	end
% 
% #ifdef self._PX4_POSIX
% 	perf_end(self.perf_accel);
% 	perf_end(self.perf_mpu);
% 	perf_end(self.perf_mag);
% #endif
% 
% 	orb_unsubscribe(self.sensors_sub);
% 	orb_unsubscribe(self.vision_sub);
% 	orb_unsubscribe(self.mocap_sub);
% 	orb_unsubscribe(self.airspeed_sub);
% 	orb_unsubscribe(self.params_sub);
% 	orb_unsubscribe(self.global_pos_sub);
end

% void AttitudeEstimatorQ:: bool
% function self = update_parameters( self,  force )
% 
% 	% bool
%     updated = force;
% 
% 	if (~updated) 
% 		% orb_check(self.params_sub, &updated);
%         updated = self.params_sub.updated;
% 	end
% 
% 	if (updated) 
% 		% parameter_update_s param_update;
% 		% orb_copy(ORB_ID(parameter_update), self.params_sub, &param_update);
% 
% % 		param_get(self.params_handles.w_acc, &self.w_accel);
% % 		param_get(self.params_handles.w_mag, &self.w_mag);
% % 		param_get(self.params_handles.w_ext_hdg, &self.w_ext_hdg);
% % 		param_get(self.params_handles.w_gyro_bias, &self.w_gyro_bias);
% % 		% float
% %         mag_decl_deg = 0.0;
% % 		param_get(self.params_handles.mag_decl, &mag_decl_deg);
% % 		update_mag_declination( radians(mag_decl_deg) );
% % 		% int32_t mag_decl_auto_int;
% % 		param_get(self.params_handles.mag_decl_auto, &mag_decl_auto_int);
% % 		self.mag_decl_auto = mag_decl_auto_int ~= 0;
% % 		% int32_t acc_comp_int;
% % 		param_get(self.params_handles.acc_comp, &acc_comp_int);
% % 		self.acc_comp = acc_comp_int ~= 0;
% % 		param_get(self.params_handles.bias_max, &self.bias_max);
% % 		param_get(self.params_handles.ext_hdg_mode, &self.ext_hdg_mode);
% % 		param_get(self.params_handles.airspeed_mode, &self.airspeed_mode);
% 	end
% end

% bool AttitudeEstimatorQ::
function [ self, output ] = init( self )

	% Rotation matrix can be easily constructed from acceleration and mag field vectors
	% 'k' is Earth Z axis (Down) unit vector in body frame
	% Vector<3>
    k = -self.accel;
	k = normalize( k );

	% 'i' is Earth X axis (North) unit vector in body frame, orthogonal with 'k'
	% Vector<3>
    i = (self.mag - (k * dot(self.mag, k) ) );
	i = normalize( i );

	% 'j' is Earth Y axis (East) unit vector in body frame, orthogonal with 'k' and 'i'
	% Vector<3>
    j = cross(k, i);

	% Fill rotation matrix
	% Matrix<3, 3>
    R = zeros(3, 3);
	R(1,:) = i; %.set_row(0, i);
	R(2,:) = j; %.set_row(1, j);
	R(3,:) = k;% .set_row(2, k);

	% Convert to quaternion
	self.q = quat_from_dcm( R );

	% Compensate for magnetic declination
	% Quaternion
    decl_rotation = quat_from_yaw( self.mag_decl );
	self.q = quat_mult(decl_rotation, self.q);

%     self.q = [-0.7147;-0.000673;-0.0003205;-0.6994];
 	self.q = normalize( self.q );
    

	if (isfinite(self.q(1)) && isfinite(self.q(2)) && ...
	    isfinite(self.q(3)) && isfinite(self.q(4)) && ...
	    ( norm( self.q ) > 0.95) && ( norm( self.q ) < 1.05) ) 
		self.inited = 1;

	else 
		self.inited = 0;
	end

	output = self.inited;
end

% bool AttitudeEstimatorQ::
function [ self, output ] = update( self, dt )

	if (~self.inited) 

        if (~self.data_good)
            output = 0;
            return;
        end

        self = init( self );
        output = 0;
		return;
	end

	% Quaternion
    q_last = self.q;

	% Angular rate of correction
	% Vector<3>
    corr  = zeros(3,1);
	% float
    spinRate = norm( self.gyro );

	if ( (self.ext_hdg_mode > 1) && self.ext_hdg_good) 
		if (self.ext_hdg_mode == 2) 
			% Vision heading correction
			% Project heading to global frame and extract XY component
			% Vector<3>
            vision_hdg_earth = quat_conjugate( self.q, self.vision_hdg );
			% float
            vision_hdg_err = wrap_pi( atan2(vision_hdg_earth(2), vision_hdg_earth(1)) );
			% Project correction to body frame
			corr = corr + quat_conjugate_inversed( self.q, [0.0; 0.0; -vision_hdg_err] ) * self.w_ext_hdg;
		end

		if (self.ext_hdg_mode == 3) 
			% Mocap heading correction
			% Project heading to global frame and extract XY component
			% Vector<3>
            mocap_hdg_earth = quat_conjugate( self.q, self.mocap_hdg );
			% float
            mocap_hdg_err = wrap_pi( atan2(mocap_hdg_earth(2), mocap_hdg_earth(1)) );
			% Project correction to body frame
			corr = corr + quat_conjugate_inversed( self.q, [0.0; 0.0; -mocap_hdg_err] ) * self.w_ext_hdg;
		end
	end

	if ( (self.ext_hdg_mode == 1) || (~self.ext_hdg_good) )
		% Magnetometer correction
		% Project mag field vector to global frame and extract XY component
		% Vector<3>
        mag_earth = quat_conjugate( self.q, self.mag );
		% float
        mag_err = wrap_pi( atan2(mag_earth(2), mag_earth(1)) - self.mag_decl);
		% float
        gainMult = 1.0;
		% const float
        fifty_dps = 0.873;

		if (spinRate > fifty_dps) 
			gainMult = min(spinRate / fifty_dps, 10.0);
		end

		% Project magnetometer correction to body frame
		corr = corr + quat_conjugate_inversed( self.q, [0.0, 0.0, -mag_err] ) * self.w_mag * gainMult;
	end

	self.q = normalize( self.q );


	% Accelerometer correction - commented out in original code
	% Project 'k' unit vector of earth frame to body frame
	% Vector<3> k = self.q.conjugate_inversed(Vector<3>(0.0, 0.0, 1.0));
	% Optimized version with dropped zeros
	% Vector<3>
    k = [ ...
		2.0 * (self.q(2) * self.q(4) - self.q(1) * self.q(3));
		2.0 * (self.q(3) * self.q(4) + self.q(1) * self.q(2));
		(self.q(1) * self.q(1) - self.q(2) * self.q(2) - self.q(3) * self.q(3) + self.q(4) * self.q(4)) ...
	];
    
    % self.acc... .normalized()
	corr = corr + cross(k, normalize(self.accel - self.pos_acc) ) * self.w_accel;

	% Gyro bias estimation
	if (spinRate < 0.175) 
		self.gyro_bias = self.gyro_bias + corr * (self.w_gyro_bias * dt);

		% for (int i = 0; i < 3; i++) 
        for i = 1:3
            self.gyro_bias(i) = constrain(self.gyro_bias(i), -self.bias_max, self.bias_max);
        end

	end

	self.rates = self.gyro + self.gyro_bias;

	% Feed forward gyro
	corr = corr + self.rates;

	% Apply correction to state
	self.q = self.q + quat_derivative( self.q, corr ) * dt;

	% Normalize quaternion
	self.q = normalize( self.q );

    if (~(isfinite(self.q(1)) && isfinite(self.q(2)) && ...
            isfinite(self.q(3)) && isfinite(self.q(4)))) 
        % Reset quaternion to last good state
        self.q = q_last;
        self.rates = zeros(3, 1);
        self.gyro_bias = zeros(3, 1);
        output = 0;
        return;
    end
    
    output = 1;
end

% void AttitudeEstimatorQ:: float 
function self = update_mag_declination( self, new_declination)
%UPDATE_MAG_DECLINATION
	% Apply initial declination or trivial rotations without changing estimation
	if (~self.inited || (abs(new_declination - self.mag_decl) < 0.0001) )
		self.mag_decl = new_declination;
	else 
		% Immediately rotate current estimation to avoid gyro bias growth
		% Quaternion
        % decl_rotation = zeros(4,1);
		decl_rotation = quat_from_yaw(new_declination - self.mag_decl);
		self.q = quat_mult( decl_rotation, self.q );
		self.mag_decl = new_declination;
	end
end

% int
% function self = attitude_estimator_q_main(int argc, char *argv[])
% 
% 	if (argc < 2)
% 		warnx('usage: attitude_estimator_q {start|stop|status}');
% 		return 1;
% 	end
% 
% 	if (~strcmp(argv[1], 'start')) 
% 
% 		if (attitude_estimator_q::instance ~= nullptr) 
% 			warnx('already running');
% 			return 1;
% 		end
% 
% 		attitude_estimator_q::instance = new AttitudeEstimatorQ;
% 
% 		if (attitude_estimator_q::instance == nullptr) 
% 			warnx('alloc failed');
% 			return 1;
% 		end
% 
% 		if (1 ~= attitude_estimator_q::instance->start()) 
% 			delete attitude_estimator_q::instance;
% 			attitude_estimator_q::instance = nullptr;
% 			warnx('start failed');
% 			return 1;
% 		end
% 
% 		return 0;
% 	end
% 
% 	if (~strcmp(argv[1], 'stop')) 
% 		if (attitude_estimator_q::instance == nullptr) 
% 			warnx('not running');
% 			return 1;
% 		end
% 
% 		delete attitude_estimator_q::instance;
% 		attitude_estimator_q::instance = nullptr;
% 		return 0;
% 	end
% 
% 	if (~strcmp(argv[1], 'status')) 
% 		if (attitude_estimator_q::instance) 
% 			attitude_estimator_q::instance->print();
% 			warnx('running');
% 			return 0;
% 
% 		else 
% 			warnx('not running');
% 			return 1;
% 		end
% 	end
% 
% 	warnx('unrecognized command');
% 	return 1;
% end

%% Math Functions
function y = constrain( x, x_min, x_max )
%CONSTRAIN
    y = max( min(x, x_max), x_min );
end

function out = normalize(in)
%NORMALIZE
    out = in ./ norm(in);
end

function out = radians(in)
%RADIANS
    out = in .* pi ./ 180;
end

function output = quat_conjugate( q, v )
%QUAT_CONJUGATE
    q0q0 = q(1) * q(1);
    q1q1 = q(2) * q(2);
    q2q2 = q(3) * q(3);
    q3q3 = q(4) * q(4);

    output = [ ...
        v(1) * (q0q0 + q1q1 - q2q2 - q3q3) + ...
        v(2) * 2.0 * (q(2) * q(3) - q(1) * q(4)) + ...
        v(3) * 2.0 * (q(1) * q(3) + q(2) * q(4)); ...
        v(1) * 2.0 * (q(2) * q(3) + q(1) * q(4)) + ...
        v(2) * (q0q0 - q1q1 + q2q2 - q3q3) + ...
        v(3) * 2.0 * (q(3) * q(4) - q(1) * q(2)); ...
        v(1) * 2.0 * (q(2) * q(4) - q(1) * q(3)) + ...
        v(2) * 2.0 * (q(1) * q(2) + q(3) * q(4)) + ...
        v(3) * (q0q0 - q1q1 - q2q2 + q3q3) ...
    ];
end

function output = quat_conjugate_inversed( q, v )
%QUAT_CONJUGATE_INVERSED
    q0q0 = q(1) * q(1);
    q1q1 = q(2) * q(2);
    q2q2 = q(3) * q(3);
    q3q3 = q(4) * q(4);

    output = [ ...
        v(1) * (q0q0 + q1q1 - q2q2 - q3q3) + ...
        v(2) * 2.0 * (q(2) * q(3) + q(1) * q(4)) + ...
        v(3) * 2.0 * (q(2) * q(4) - q(1) * q(3)); ...
        v(1) * 2.0 * (q(2) * q(3) - q(1) * q(4)) + ...
        v(2) * (q0q0 - q1q1 + q2q2 - q3q3) + ...
        v(3) * 2.0 * (q(3) * q(4) + q(1) * q(2)); ...
        v(1) * 2.0 * (q(2) * q(4) + q(1) * q(3)) + ...
        v(2) * 2.0 * (q(3) * q(4) - q(1) * q(2)) + ...
        v(3) * (q0q0 - q1q1 - q2q2 + q3q3) ...
    ];
end

function R  = quat_to_dcm( data )
%QUAT_TO_DCM Convert quaternion to DCM
%   From https://github.com/PX4/Firmware/blob/master/src/lib/mathlib/math/Quaternion.hpp
    aSq = data(1) * data(1);
    bSq = data(2) * data(2);
    cSq = data(3) * data(3);
    dSq = data(4) * data(4);
    R = zeros(3,3);
    R(1,1) = aSq + bSq - cSq - dSq;
    R(1,2) = 2.0 * ( data(2) * data(3) - data(1) * data(4) );
    R(1,3) = 2.0 * ( data(1) * data(3) + data(2) * data(4) );
    R(2,1) = 2.0 * ( data(2) * data(3) + data(1) * data(4) );
    R(2,2) = aSq - bSq + cSq - dSq;
    R(2,3) = 2.0 * ( data(3) * data(4) - data(1) * data(2) );
    R(3,1) = 2.0 * ( data(2) * data(4) - data(1) * data(3) );
    R(3,2) = 2.0 * ( data(1) * data(2) + data(3) * data(4) );
    R(3,3) = aSq - bSq - cSq + dSq;
end

function q = quat_from_yaw( yaw )
%QUAT_FROM_YAW
    q = zeros(4,1);
    q(1) = cos(yaw / 2.0);
    q(2) = 0.0;
    q(3) = 0.0;
    q(4) = sin(yaw / 2.0);
end

function data  = quat_from_dcm( dcm )
%QUAT_FROM_DCM Convert DCM to quaternion
%   From https://github.com/PX4/Firmware/blob/master/src/lib/mathlib/math/Quaternion.hpp
    data = zeros(4,1);
    tr = dcm(1,1) + dcm(2,2) + dcm(3,3);
    if (tr > 0.0)
        s = sqrt(tr + 1.0);
        data(1) = s * 0.5;
        s = 0.5 / s;
        data(2) = (dcm(3,2) - dcm(2,3) ) * s;
        data(3) = (dcm(1,3) - dcm(3,1) ) * s;
        data(4) = (dcm(2,1) - dcm(1,2) ) * s;
    else
        % Find maximum diagonal element in dcm
        % store index in dcm_i
        dcm_i = 1;
        for i = 2:3 % (int i = 1; i < 3; i++)
            if ( dcm(i,i) > dcm(dcm_i,dcm_i) )
                dcm_i = i;
            end
        end
        dcm_j = rem( ( (dcm_i-1) + 1), 3) + 1;
        dcm_k = rem( ( (dcm_i-1) + 2), 3) + 1;
        s = sqrt( (dcm(dcm_i, dcm_i) - dcm(dcm_j, dcm_j) - ...
            dcm(dcm_k,dcm_k)) + 1.0 );
        data(dcm_i + 1) = s * 0.5;
        s = 0.5 / s;
        data(dcm_j + 1) = ( dcm(dcm_i,dcm_j) + dcm(dcm_j,dcm_i) ) * s;
        data(dcm_k + 1) = ( dcm(dcm_k,dcm_i) + dcm(dcm_i,dcm_k) ) * s;
        data(1) = ( dcm(dcm_k,dcm_j) - dcm(dcm_j,dcm_k) ) * s;
    end
end

function [ qOut ] = quat_mult( q1, q2 )
%QUATMULT Multiply quatrenion q1 by quaternion q2
%   Written by: J.X.J. Bannwarth, 28/03/2017
    
    % Normal quaternion
    qOut = zeros(4,1);
    qOut(1,1) = q1(1) * q2(1) - q1(2) * q2(2) - q1(3) * q2(3) - q1(4) * q2(4);
    qOut(2,1) = q1(1) * q2(2) + q1(2) * q2(1) + q1(3) * q2(4) - q1(4) * q2(3);
    qOut(3,1) = q1(1) * q2(3) - q1(2) * q2(4) + q1(3) * q2(1) + q1(4) * q2(2);
    qOut(4,1) = q1(1) * q2(4) + q1(2) * q2(3) - q1(3) * q2(2) + q1(4) * q2(1);
end

% Check order of Q elements
% const Vector<3> &
function quat_deriv = quat_derivative( q, w )
%QUAT_DERIVATIVE
    Q = [ ...
    q(1), -q(2), -q(3), -q(4);
    q(2),  q(1), -q(4),  q(3);
    q(3),  q(4),  q(1), -q(2);
    q(4), -q(3),  q(2),  q(1) ];
    v = [0.0; w(1); w(2); w(3) ];
    quat_deriv = Q * v * 0.5;
end

% float
function output = get_mag_declination(lat, lon)
%GET_MAG_DECLINATION
% If the values exceed valid ranges, return zero as default
% as we have no way of kself.nowing what the closest real value
% would be.
    SAMPLING_RES     =   10.0;
    SAMPLING_MAX_LAT =   60.0;
    SAMPLING_MIN_LAT = - 60.0;
    SAMPLING_MIN_LON = -180.0;
    SAMPLING_MAX_LON =  180.0;

    if (lat < -90.0 || lat > 90.0 || ...
        lon < -180.0 || lon > 180.0)
        output = 0.0;
        return;
    end

	% Round down to nearest sampling resolution
	min_lat = floor((lat / SAMPLING_RES) * SAMPLING_RES);
	min_lon = floor((lon / SAMPLING_RES) * SAMPLING_RES);

	% Find index of nearest low sampling point
	[min_lat_index, min_lat] = get_lookup_table_index( min_lat, SAMPLING_MIN_LAT, SAMPLING_MAX_LAT);
	[min_lon_index, min_lon] = get_lookup_table_index( min_lon, SAMPLING_MIN_LON, SAMPLING_MAX_LON);

	declination_sw = get_lookup_table_val(min_lat_index, min_lon_index);
	declination_se = get_lookup_table_val(min_lat_index, min_lon_index + 1);
	declination_ne = get_lookup_table_val(min_lat_index + 1, min_lon_index + 1);
	declination_nw = get_lookup_table_val(min_lat_index + 1, min_lon_index);

	% Perform bilinear interpolation on the four grid corners
	lat_scale = constrain( (lat - min_lat) / SAMPLING_RES, 0.0, 1.0 );
	lon_scale = constrain( (lon - min_lon) / SAMPLING_RES, 0.0, 1.0 );

	declination_min = lon_scale * (declination_se - declination_sw) + declination_sw;
	declination_max = lon_scale * (declination_ne - declination_nw) + declination_nw;

	output = lat_scale * (declination_max - declination_min) + declination_min;
end

% unsigned
function [ output, val ] = get_lookup_table_index( val, min, max)
%GET_LOOKUP_TABLE_INDEX
%   for the rare case of hitting the bounds exactly
%   the rounding logic wouldn't fit, so enforce it.
    SAMPLING_RES = 10.0;

    % Limit to table bounds - required for maxima even when table spans full globe range
    if ( val < min )
        val = min;
    end

    % Limit to (table bounds - 1) because bilinear interpolation requires checking (index + 1)
    if ( val > max )
        val = max - SAMPLING_RES;
    end

    output = floor( ( -(min) + val )  / SAMPLING_RES );
end

% float
function output = get_lookup_table_val(lat_index, lon_index)
%GET_LOOKUP_TABLE_VAL
declination_table = [ ...
    47, 45, 44, 43, 41, 40, 38, 36, 33, 28, 23, 16, 10, 4, -1, -5, -9, -14, -19, -26, -33, -41, -48, -55, -61, -67, -71, -74, -75, -72, -61, -23, 23, 41, 46, 47, 47 ;
    30, 30, 30, 30, 30, 29, 29, 29, 27, 23, 18, 11, 3, -3, -9, -12, -15, -17, -21, -26, -32, -39, -46, -51, -55, -57, -56, -52, -44, -31, -14, 1, 13, 21, 26, 29, 30 ;
    22, 22, 22, 22, 22, 22, 22, 22, 21, 18, 13, 5, -3, -11, -17, -20, -21, -22, -23, -25, -29, -35, -40, -44, -45, -44, -39, -31, -21, -11, -3, 3, 9, 14, 18, 20, 22 ;
    16, 17, 17, 17, 17, 16, 16, 16, 15, 13, 8, 0, -9, -17, -22, -24, -25, -24, -22, -20, -21, -24, -29, -31, -31, -28, -23, -16, -9, -3, 0, 4, 7, 10, 13, 15, 16 ;
    12, 13, 13, 13, 13, 13, 12, 12, 11, 9, 3, -4, -13, -19, -23, -24, -24, -21, -17, -12, -9, -10, -14, -17, -18, -16, -12, -8, -3, 0, 1, 3, 5, 8, 10, 12, 12 ;
    10, 10, 10, 10, 10, 10, 10, 9, 8, 5, 0, -7, -15, -20, -22, -22, -19, -15, -10, -5, -2, -1, -4, -7, -8, -8, -6, -3, 0, 0, 1, 2, 4, 6, 8, 10, 10 ;
    9, 9, 9, 9, 9, 9, 8, 8, 7, 3, -2, -9, -15, -19, -20, -17, -13, -9, -5, -2, 0, 1, 0, -2, -3, -4, -3, -2, 0, 0, 0, 1, 2, 5, 7, 8, 9 ;
    8, 8, 8, 9, 9, 9, 8, 7, 5, 1, -3, -10, -15, -17, -17, -14, -10, -5, -2, 0, 1, 2, 2, 0, -1, -1, -1, -1, 0, 0, 0, 0, 0, 3, 5, 7, 8 ;
    8, 8, 9, 9, 10, 10, 9, 8, 5, 0, -5, -11, -15, -16, -15, -11, -7, -3, -1, 0, 2, 3, 3, 1, 0, 0, 0, 0, 0, -1, -2, -3, -2, 0, 3, 6, 8 ;
    6, 8, 10, 11, 12, 12, 11, 9, 5, 0, -7, -12, -15, -15, -13, -10, -6, -3, 0, 1, 3, 4, 4, 3, 2, 1, 1, 0, -1, -3, -5, -6, -5, -3, 0, 3, 6 ;
    5, 8, 11, 13, 14, 15, 13, 10, 5, -1, -9, -14, -16, -16, -13, -10, -6, -3, 0, 2, 3, 5, 5, 5, 5, 4, 3, 1, -1, -4, -7, -9, -8, -6, -2, 1, 5 ;
    3, 8, 12, 15, 17, 17, 16, 12, 5, -3, -12, -18, -20, -19, -16, -12, -8, -4, 0, 2, 4, 7, 8, 9, 10, 9, 7, 3, -1, -6, -10, -12, -11, -9, -5, 0, 3 ;
    3, 8, 13, 16, 19, 20, 19, 14, 4, -7, -18, -24, -26, -24, -21, -16, -11, -6, -2, 2, 6, 10, 13, 15, 17, 16, 13, 7, 0, -7, -13, -15, -14, -11, -6, -1, 3 ];
	output = declination_table(lat_index, lon_index);
end

function bearing = wrap_pi(bearing)
%WRAP_PI
    % value is inf or NaN
    if (~isfinite(bearing))
        return
    end

    c = 0;

    while (bearing >= 3.14159265)
        bearing = bearing - 6.28318531;

        if (c > 3)
            bearing = nan;
            return
        end
        c = c + 1;
    end

    c = 0;

    while (bearing < -3.14159265)
        bearing = bearing + 6.28318531;

        if (c > 3)
            bearing = nan;
            return
        end
        c = c + 1;
    end
end

%% 2nd Order Low Pass Filter
%void LowPassFilter2p:: float float
function lp2p = lp2p_set_cutoff_frequency( lp2p, sample_freq, cutoff_freq )
	lp2p.cutoff_freq = cutoff_freq;

    M_PI_F = 3.14159265358979323846;
    
    if (lp2p.cutoff_freq <= 0.0)
        % no filtering
        return;
    end

	fr = sample_freq / lp2p.cutoff_freq;
	ohm = tan( M_PI_F / fr );
	c = 1.0 + 2.0 * cos( M_PI_F / 4.0 ) * ohm + ohm * ohm;
	lp2p.b0 = ohm * ohm / c;
	lp2p.b1 = 2.0 * lp2p.b0;
	lp2p.b2 = lp2p.b0;
	lp2p.a1 = 2.0 * (ohm * ohm - 1.0) / c;
	lp2p.a2 = (1.0 - 2.0 * cos( M_PI_F / 4.0 ) * ohm + ohm * ohm) / c;
end

% float LowPassFilter2p::
function [ lp2p, output ] = lp2p_apply( lp2p, sample )
    if ( lp2p.cutoff_freq <= 0.0 )
        % no filtering
        output = sample;
        return;
    end

	% do the filtering
	delay_element_0 = sample - lp2p.delay_element_1 * lp2p.a1 - lp2p.delay_element_2 * lp2p.a2;

    if (~isfinite(delay_element_0))
        % don't allow bad values to propagate via the filter
        delay_element_0 = sample;
    end

	output = delay_element_0 * lp2p.b0 + ...
        lp2p.delay_element_1 * lp2p.b1 + lp2p.delay_element_2 * lp2p.b2;

	lp2p.delay_element_2 = lp2p.delay_element_1;
	lp2p.delay_element_1 = delay_element_0;

	% return the value.  Should be no need to check limits
% 	return output;
end

% float LowPassFilter2p::
% function [ lp2p, output ] = lp2p_reset( lp2p, sample )
% 	dval = sample / (lp2p.b0 + lp2p.b1 + lp2p.b2);
% 	lp2p.delay_element_1 = dval;
% 	lp2p.delay_element_2 = dval;
% 	[ lp2p, output ] = lp2p_apply( lp2p, sample );
% end
